simulink model "CardiacAI_v2"  (R2020b)
settings: Solver=FixedStepAuto  StartTime=0.0  StopTime=10.0  RelTol=1e-3
values from neighbouring files (symbols this model uses):
  HEALTHY_img_resized_flipped = flip(HEALTHY_img_resized,2)    [img_resize.m]
  UNHEALTHY_img_resized_flipped = flip(UNHEALTHY_img_resized,2)    [img_resize.m]
undefined symbols (not defined in the file or in its folder): DiscIntNeverNeededParam
libraries: androiduilib x4, androidaudiovideolib x3
settings Model: Creator=mesutguven  LastModifiedBy=mesutguven
settings OptimizationCC: EnhancedBackFolding=on  PassReuseOutputArgsAs=Individual arguments  ZeroExternalMemoryAtStartup=off  ZeroInternalMemoryAtStartup=off  MaxStackSize=64  OptimizeBlockOrder=speed  DifferentSizesBufferReuse=on  OptimizationCustomize=off  EfficientTunableParamExpr=on
settings DebuggingCC: ParameterTunabilityLossMsg=error
settings HardwareCC: ProdBitPerPointer=32  ProdBitPerSizeT=32  ProdBitPerPtrDiffT=32  ProdLargestAtomicInteger=Long  ProdLargestAtomicFloat=Double  ProdWordSize=32  ProdHWDeviceType=ARM Compatible->ARM Cortex  UseEmbeddedCoderFeatures=off  UseSimulinkCoderFeatures=off
settings SFSimCC: MATLABDynamicMemAlloc=off
settings RTWCC: Description=Embedded Coder  SystemTargetFile=ert.tlc  HardwareBoard=Android Device  TLCOptions="-aInlineSetEventsForThisBaseRateFcn=TLC_FALSE -aSuppressMultiTaskScheduler=TLC_FALSE  -aRateBasedStepFcn=0"  TemplateMakefile=ert_default_tmf  RTWVerbose=off  Toolchain=Android SDK/NDK Tools
settings CodeAppCC: ForceParamTrailComments=on  IgnoreCustomStorageClasses=off  OperatorAnnotations=on  SimulinkDataObjDesc=on  SFDataObjDesc=on  InsertBlockDesc=on
settings ERTTargetCC: SupportNonInlinedSFcns=on

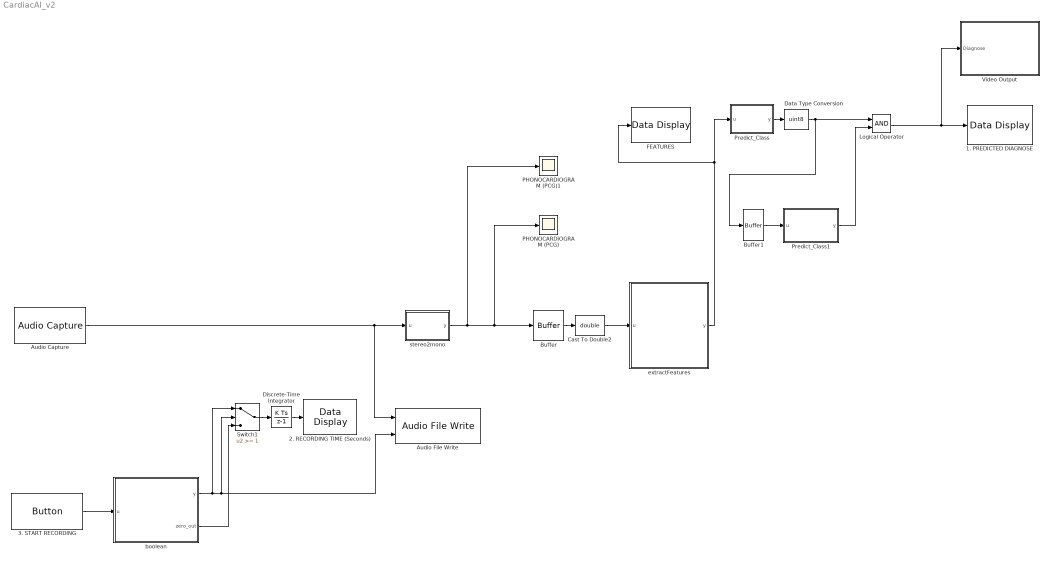
== system CardiacAI_v2 ==
  " PHONOCARDIOGRAM (PCG)" : Scope
  " PHONOCARDIOGRAM (PCG)1" : Scope
  " boolean" : MATLAB Function  TreatAsAtomicUnit=on
  " stereo2mono" : MATLAB Function  TreatAsAtomicUnit=on
  1. PREDICTED DIAGNOSE : androiduilib/Data Display  DataDisplayId=CardiacAI_v2/1._PREDICTED_DIAGNOSE  Format=Integer  Precision=6  SimulateUsing=Code generation  blockPlatform=Android
      settings: SourceProductName=Simulink Support Package for Android Devices
  2. RECORDING TIME (Seconds) : androiduilib/Data Display  DataDisplayId=CardiacAI_v2/2._RECORDING_TIME_(Seconds)  Format=Float  Precision=2  SimulateUsing=Code generation  blockPlatform=Android
      settings: SourceProductBaseCode=ANDROID
  3. START RECORDING : androiduilib/Button  ButtonState=Not pressed  ButtonId=CardiacAI_v2/3._START_RECORDING  State=off  SampleTime=0.1  BlockPlatform=Android
      settings: SourceProductBaseCode=ANDROID
  Audio Capture : androidaudiovideolib/Audio Capture  SampleFreq=44100  FrameSize=4410  SampleTime=0.1  SimulateUsing=Code generation  DeviceStr=0  QueueDuration=0  BlockPlatform=Android  AudioSamplingFreq=44100
      settings: SourceProductName=Simulink Support Package for Android Devices
  Audio File Write : androidaudiovideolib/Audio File Write  FileName=Recorded_PCG_Signal  FileType=wav  AudioSamplingFreq=44100  RecordTimeControl=Input port  MaxRecordTime=60  BitRate=128  AudioFileWriteId=CardiacAI_v2/Audio_File_Write  SimulateUsing=Code generation
      settings: SourceProductBaseCode=ANDROID
  Buffer : Buffer  N=220500  OutputFrames=off
  Buffer1 : Buffer  N=2  OutputFrames=off
  Cast To Double2 : DataTypeConversion  OutDataTypeStr=double
  Data Type Conversion : DataTypeConversion  OutDataTypeStr=uint8
  Discrete-Time Integrator : DiscreteIntegrator  SampleTime=-1  ICPrevOutput=DiscIntNeverNeededParam  ICPrevScaledInput=DiscIntNeverNeededParam
  FEATURES : androiduilib/Data Display  DataDisplayId=CardiacAI_v2/FEATURES  Format=Float  Precision=6  SimulateUsing=Code generation  blockPlatform=Android
      settings: SourceProductBaseCode=ANDROID
  Logical Operator : Logic  AllPortsSameDT=off  OutDataTypeStr=boolean
  Predict_Class : MATLAB Function  TreatAsAtomicUnit=on
  Predict_Class1 : MATLAB Function  TreatAsAtomicUnit=on
  Switch1 : Switch  Threshold=1
  Video Output : Subsystem
  extractFeatures : MATLAB Function  TreatAsAtomicUnit=on
  wires:
  Cast To Double2/1 -> extractFeatures/1(u)
  extractFeatures/1(y) -> Predict_Class/1(u), FEATURES/1
  Data Type Conversion/1 -> Logical Operator/1, Buffer1/1
  Buffer/1 -> Cast To Double2/1
  Predict_Class/1(y) -> Data Type Conversion/1
  Audio Capture/1 -> Audio File Write/1, " stereo2mono"/1(u)
  " stereo2mono"/1(y) -> " PHONOCARDIOGRAM (PCG)1"/1, Buffer/1, " PHONOCARDIOGRAM (PCG)"/1
  " boolean"/2(zero_out) -> Switch1/3
  3. START RECORDING/1 -> " boolean"/1(u)
  " boolean"/1(y) -> Switch1/1, Switch1/2, Audio File Write/2
  Discrete-Time Integrator/1 -> 2. RECORDING TIME (Seconds)/1
  Switch1/1 -> Discrete-Time Integrator/1
  Buffer1/1 -> Predict_Class1/1(u)
  Predict_Class1/1(y) -> Logical Operator/2
  Logical Operator/1 -> Video Output/1(Diagnose), 1. PREDICTED DIAGNOSE/1

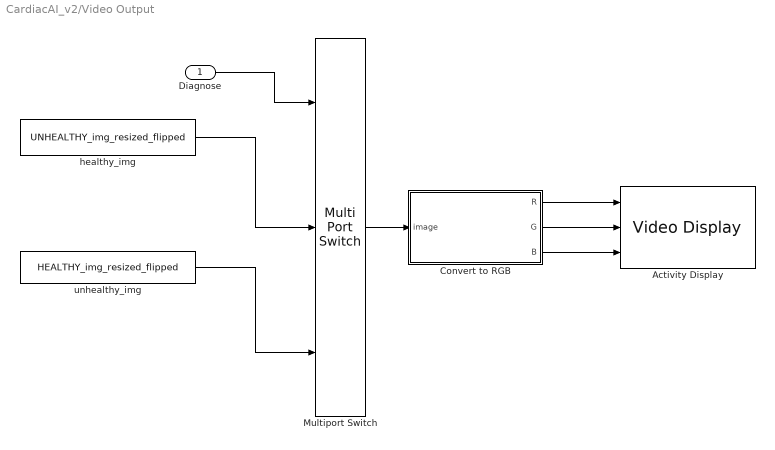
== system CardiacAI_v2/Video Output ==
  Diagnose : Inport
  Activity Display : androidaudiovideolib/Video Display  BlockPlatform=Android
      settings: SourceProductName=Simulink Support Package for Android Devices
  Convert to RGB : MATLAB Function  TreatAsAtomicUnit=on
  Multiport Switch : MultiPortSwitch  Inputs=2  DiagnosticForDefault=None
  healthy_img : Constant  Value=UNHEALTHY_img_resized_flipped  VectorParams1D=off
  unhealthy_img : Constant  Value=HEALTHY_img_resized_flipped  VectorParams1D=off
  wires:
  Convert to RGB/3(B) -> Activity Display/3
  unhealthy_img/1 -> Multiport Switch/3
  Diagnose/1 -> Multiport Switch/1
  Convert to RGB/1(R) -> Activity Display/1
  Multiport Switch/1 -> Convert to RGB/1(image)
  Convert to RGB/2(G) -> Activity Display/2
  healthy_img/1 -> Multiport Switch/2

== matlab function CardiacAI_v2/ boolean ==
  data: u input; y output; zero_out output
function [y, zero_out] = boolean(u)

y = double(u);

zero_out = 0;
end

== matlab function CardiacAI_v2/Predict_Class ==
  data: u input; y output
function y= Predict_Class(u)

persistent mdl;

   if isempty(mdl)
   
       mdl = loadLearnerForCoder('TrainedEnsembleModel_FeatSel.mat');
   
   end
   
 predicted_class = predict (mdl, u);   
   
  if isequal(predicted_class {1}, 'Normal')
     
   y = 0;
 else
   y = 1;
 
 end

end

== matlab function CardiacAI_v2/ stereo2mono ==
  data: u input; y output
function y = strero2mono(u)

y = u(:,1);

end

== matlab function CardiacAI_v2/extractFeatures ==
  data: u input; y output

function y  = exractFeatures(u)

desiredFs = 44100;

window_length = 5;    

current_signal = u;
[~,c] = size (current_signal);
        if c ~= 1
          signal = current_signal';
          
        else
          signal = current_signal;
       end

c_signal = signal/32857;

features = zeros (1,15);
       

        % 9 Calculate kurtosis of the signal values
        features(1) = kurtosis(c_signal);

        % 12, 13, 14 Extract features from the power spectrum
        [maxfreq] = dominant_frequency_features(c_signal, desiredFs, 256, 0);
        
        features(2) = maxfreq;    % 12
        
        % Extract Mel-frequency cepstral coefficients
        Tw = window_length*1000;% analysis frame duration (ms)
        Ts = 10;                % analysis frame shift (ms)
        alpha = 0.97;           % preemphasis coefficient
        M = 20;                 % number of filterbank channels 
        C = 12;                 % number of cepstral coefficients
        L = 22;                 % cepstral sine lifter parameter
        LF = 5;                 % lower frequency limit (Hz)
        HF = 500;               % upper frequency limit (Hz)

       [MFCCs, ~, ~] = mfcc(c_signal, desiredFs, Tw, Ts, alpha, @hamming, [LF HF], M, C+1, L);
        
        features(3) = MFCCs(1);   % 15 
        features(4) = MFCCs(2);   % 16
        features(5) = MFCCs(3);   % 17
        features(6) = MFCCs(4);   % 18
        features(7) = MFCCs(5);   % 19
        features(8) = MFCCs(6);   % 20
        features(9) = MFCCs(7);   % 21
        features(10) = MFCCs(8);  % 22
        features(11) = MFCCs(9);  % 23
        features(12) = MFCCs(10); % 24
        features(13) = MFCCs(11); % 25
        features(14) = MFCCs(12); % 26
        features(15) = MFCCs(13); % 27
        
y = features;

end

== matlab function CardiacAI_v2/Video Output/Convert to RGB ==
  data: image input; R output; G output; B output
function [R,G,B] = deconcatenate(image)
% deconcatenate - Extract Red, Green and Blue channels from a RGB image. 

% Copyright 2017 The MathWorks, Inc.

R = image(:,:,1);
G = image(:,:,2);
B = image(:,:,3);

== matlab function CardiacAI_v2/Predict_Class1 ==
  data: u input; y output
function y= Predict_Class_1(u)

if  u(1)*u(2)==0
    mult=0;
else
    mult=1;
end
    y=mult;
end
